simulink model "Dijkstra_Optimization_2"  (R2015b)
settings: Solver=FixedStepDiscrete  SolverMode=SingleTasking  StartTime=0.0  StopTime=10e-5  RelTol=1e-3
libraries: shlslibv1 x995
(part 1 of 6)
settings Model: synDspstartup=OK  Creator=irupawal  LastModifiedBy=vrames13
settings DataIOCC: SaveOutput=off  SignalLogging=off  SaveTime=off
settings OptimizationCC: DefaultParameterBehavior=Inlined
settings DebuggingCC: AlgebraicLoopMsg=error  InheritedTsInSrcMsg=none

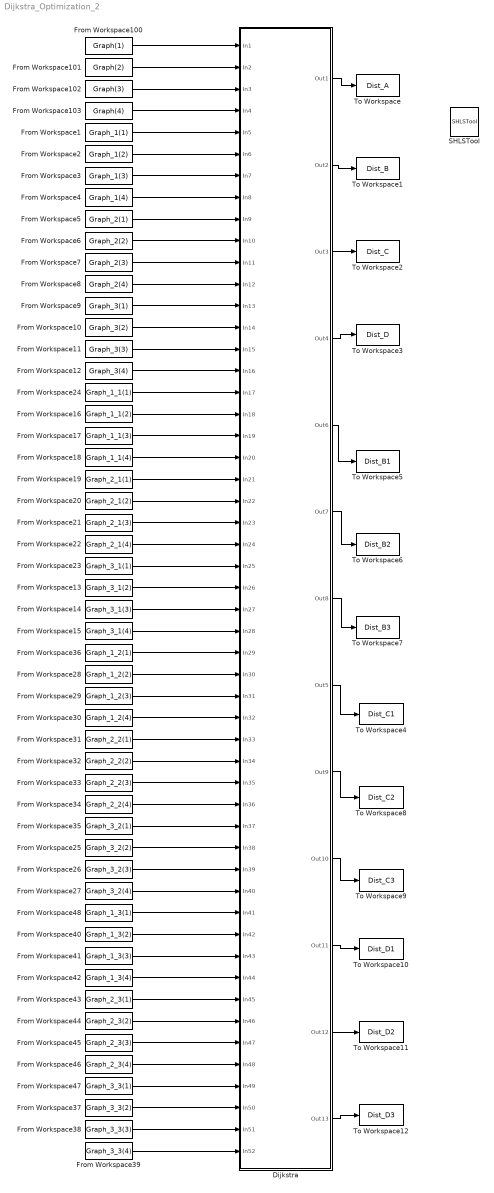
== system Dijkstra_Optimization_2 ==
  Dijkstra : Subsystem
  From Workspace1 : FromWorkspace  VariableName=Graph_1(1)  SampleTime=1/(16e6)  Interpolate=off  OutputAfterFinalValue=Holding final value
  From Workspace10 : FromWorkspace  VariableName=Graph_3(2)  SampleTime=1/(16e6)  Interpolate=off  OutputAfterFinalValue=Holding final value
  From Workspace100 : FromWorkspace  VariableName=Graph(1)  SampleTime=1/(16e6)  Interpolate=off  OutputAfterFinalValue=Holding final value
  From Workspace101 : FromWorkspace  VariableName=Graph(2)  SampleTime=1/(16e6)  Interpolate=off  OutputAfterFinalValue=Holding final value
  From Workspace102 : FromWorkspace  VariableName=Graph(3)  SampleTime=1/(16e6)  Interpolate=off  OutputAfterFinalValue=Holding final value
  From Workspace103 : FromWorkspace  VariableName=Graph(4)  SampleTime=1/(16e6)  Interpolate=off  OutputAfterFinalValue=Holding final value
  From Workspace11 : FromWorkspace  VariableName=Graph_3(3)  SampleTime=1/(16e6)  Interpolate=off  OutputAfterFinalValue=Holding final value
  From Workspace12 : FromWorkspace  VariableName=Graph_3(4)  SampleTime=1/(16e6)  Interpolate=off  OutputAfterFinalValue=Holding final value
  From Workspace13 : FromWorkspace  VariableName=Graph_3_1(2)  SampleTime=1/(16e6)  Interpolate=off  OutputAfterFinalValue=Holding final value
  From Workspace14 : FromWorkspace  VariableName=Graph_3_1(3)  SampleTime=1/(16e6)  Interpolate=off  OutputAfterFinalValue=Holding final value
  From Workspace15 : FromWorkspace  VariableName=Graph_3_1(4)  SampleTime=1/(16e6)  Interpolate=off  OutputAfterFinalValue=Holding final value
  From Workspace16 : FromWorkspace  VariableName=Graph_1_1(2)  SampleTime=1/(16e6)  Interpolate=off  OutputAfterFinalValue=Holding final value
  From Workspace17 : FromWorkspace  VariableName=Graph_1_1(3)  SampleTime=1/(16e6)  Interpolate=off  OutputAfterFinalValue=Holding final value
  From Workspace18 : FromWorkspace  VariableName=Graph_1_1(4)  SampleTime=1/(16e6)  Interpolate=off  OutputAfterFinalValue=Holding final value
  From Workspace19 : FromWorkspace  VariableName=Graph_2_1(1)  SampleTime=1/(16e6)  Interpolate=off  OutputAfterFinalValue=Holding final value
  From Workspace2 : FromWorkspace  VariableName=Graph_1(2)  SampleTime=1/(16e6)  Interpolate=off  OutputAfterFinalValue=Holding final value
  From Workspace20 : FromWorkspace  VariableName=Graph_2_1(2)  SampleTime=1/(16e6)  Interpolate=off  OutputAfterFinalValue=Holding final value
  From Workspace21 : FromWorkspace  VariableName=Graph_2_1(3)  SampleTime=1/(16e6)  Interpolate=off  OutputAfterFinalValue=Holding final value
  From Workspace22 : FromWorkspace  VariableName=Graph_2_1(4)  SampleTime=1/(16e6)  Interpolate=off  OutputAfterFinalValue=Holding final value
  From Workspace23 : FromWorkspace  VariableName=Graph_3_1(1)  SampleTime=1/(16e6)  Interpolate=off  OutputAfterFinalValue=Holding final value
  From Workspace24 : FromWorkspace  VariableName=Graph_1_1(1)  SampleTime=1/(16e6)  Interpolate=off  OutputAfterFinalValue=Holding final value
  From Workspace25 : FromWorkspace  VariableName=Graph_3_2(2)  SampleTime=1/(16e6)  Interpolate=off  OutputAfterFinalValue=Holding final value
  From Workspace26 : FromWorkspace  VariableName=Graph_3_2(3)  SampleTime=1/(16e6)  Interpolate=off  OutputAfterFinalValue=Holding final value
  From Workspace27 : FromWorkspace  VariableName=Graph_3_2(4)  SampleTime=1/(16e6)  Interpolate=off  OutputAfterFinalValue=Holding final value
  From Workspace28 : FromWorkspace  VariableName=Graph_1_2(2)  SampleTime=1/(16e6)  Interpolate=off  OutputAfterFinalValue=Holding final value
  From Workspace29 : FromWorkspace  VariableName=Graph_1_2(3)  SampleTime=1/(16e6)  Interpolate=off  OutputAfterFinalValue=Holding final value
  From Workspace3 : FromWorkspace  VariableName=Graph_1(3)  SampleTime=1/(16e6)  Interpolate=off  OutputAfterFinalValue=Holding final value
  From Workspace30 : FromWorkspace  VariableName=Graph_1_2(4)  SampleTime=1/(16e6)  Interpolate=off  OutputAfterFinalValue=Holding final value
  From Workspace31 : FromWorkspace  VariableName=Graph_2_2(1)  SampleTime=1/(16e6)  Interpolate=off  OutputAfterFinalValue=Holding final value
  From Workspace32 : FromWorkspace  VariableName=Graph_2_2(2)  SampleTime=1/(16e6)  Interpolate=off  OutputAfterFinalValue=Holding final value
  From Workspace33 : FromWorkspace  VariableName=Graph_2_2(3)  SampleTime=1/(16e6)  Interpolate=off  OutputAfterFinalValue=Holding final value
  From Workspace34 : FromWorkspace  VariableName=Graph_2_2(4)  SampleTime=1/(16e6)  Interpolate=off  OutputAfterFinalValue=Holding final value
  From Workspace35 : FromWorkspace  VariableName=Graph_3_2(1)  SampleTime=1/(16e6)  Interpolate=off  OutputAfterFinalValue=Holding final value
  From Workspace36 : FromWorkspace  VariableName=Graph_1_2(1)  SampleTime=1/(16e6)  Interpolate=off  OutputAfterFinalValue=Holding final value
  From Workspace37 : FromWorkspace  VariableName=Graph_3_3(2)  SampleTime=1/(16e6)  Interpolate=off  OutputAfterFinalValue=Holding final value
  From Workspace38 : FromWorkspace  VariableName=Graph_3_3(3)  SampleTime=1/(16e6)  Interpolate=off  OutputAfterFinalValue=Holding final value
  From Workspace39 : FromWorkspace  VariableName=Graph_3_3(4)  SampleTime=1/(16e6)  Interpolate=off  OutputAfterFinalValue=Holding final value
  From Workspace4 : FromWorkspace  VariableName=Graph_1(4)  SampleTime=1/(16e6)  Interpolate=off  OutputAfterFinalValue=Holding final value
  From Workspace40 : FromWorkspace  VariableName=Graph_1_3(2)  SampleTime=1/(16e6)  Interpolate=off  OutputAfterFinalValue=Holding final value
  From Workspace41 : FromWorkspace  VariableName=Graph_1_3(3)  SampleTime=1/(16e6)  Interpolate=off  OutputAfterFinalValue=Holding final value
  From Workspace42 : FromWorkspace  VariableName=Graph_1_3(4)  SampleTime=1/(16e6)  Interpolate=off  OutputAfterFinalValue=Holding final value
  From Workspace43 : FromWorkspace  VariableName=Graph_2_3(1)  SampleTime=1/(16e6)  Interpolate=off  OutputAfterFinalValue=Holding final value
  From Workspace44 : FromWorkspace  VariableName=Graph_2_3(2)  SampleTime=1/(16e6)  Interpolate=off  OutputAfterFinalValue=Holding final value
  From Workspace45 : FromWorkspace  VariableName=Graph_2_3(3)  SampleTime=1/(16e6)  Interpolate=off  OutputAfterFinalValue=Holding final value
  From Workspace46 : FromWorkspace  VariableName=Graph_2_3(4)  SampleTime=1/(16e6)  Interpolate=off  OutputAfterFinalValue=Holding final value
  From Workspace47 : FromWorkspace  VariableName=Graph_3_3(1)  SampleTime=1/(16e6)  Interpolate=off  OutputAfterFinalValue=Holding final value
  From Workspace48 : FromWorkspace  VariableName=Graph_1_3(1)  SampleTime=1/(16e6)  Interpolate=off  OutputAfterFinalValue=Holding final value
  From Workspace5 : FromWorkspace  VariableName=Graph_2(1)  SampleTime=1/(16e6)  Interpolate=off  OutputAfterFinalValue=Holding final value
  From Workspace6 : FromWorkspace  VariableName=Graph_2(2)  SampleTime=1/(16e6)  Interpolate=off  OutputAfterFinalValue=Holding final value
  From Workspace7 : FromWorkspace  VariableName=Graph_2(3)  SampleTime=1/(16e6)  Interpolate=off  OutputAfterFinalValue=Holding final value
  From Workspace8 : FromWorkspace  VariableName=Graph_2(4)  SampleTime=1/(16e6)  Interpolate=off  OutputAfterFinalValue=Holding final value
  From Workspace9 : FromWorkspace  VariableName=Graph_3(1)  SampleTime=1/(16e6)  Interpolate=off  OutputAfterFinalValue=Holding final value
  SHLSTool : shlslibv1/SHLSTool  synBlockType=tool  syn_dsp_mode=FPGA
  To Workspace : ToWorkspace  VariableName=Dist_A  SaveFormat=Timeseries  SampleTime=-1
  To Workspace1 : ToWorkspace  VariableName=Dist_B  SaveFormat=Timeseries  SampleTime=-1
  To Workspace10 : ToWorkspace  VariableName=Dist_D1  SaveFormat=Timeseries  SampleTime=-1
  To Workspace11 : ToWorkspace  VariableName=Dist_D2  SaveFormat=Timeseries  SampleTime=-1
  To Workspace12 : ToWorkspace  VariableName=Dist_D3  SaveFormat=Timeseries  SampleTime=-1
  To Workspace2 : ToWorkspace  VariableName=Dist_C  SaveFormat=Timeseries  SampleTime=-1
  To Workspace3 : ToWorkspace  VariableName=Dist_D  SaveFormat=Timeseries  SampleTime=-1
  To Workspace4 : ToWorkspace  VariableName=Dist_C1  SaveFormat=Timeseries  SampleTime=-1
  To Workspace5 : ToWorkspace  VariableName=Dist_B1  SaveFormat=Timeseries  SampleTime=-1
  To Workspace6 : ToWorkspace  VariableName=Dist_B2  SaveFormat=Timeseries  SampleTime=-1
  To Workspace7 : ToWorkspace  VariableName=Dist_B3  SaveFormat=Timeseries  SampleTime=-1
  To Workspace8 : ToWorkspace  VariableName=Dist_C2  SaveFormat=Timeseries  SampleTime=-1
  To Workspace9 : ToWorkspace  VariableName=Dist_C3  SaveFormat=Timeseries  SampleTime=-1
  wires:
  From Workspace100/1 -> Dijkstra/1(In1)
  From Workspace101/1 -> Dijkstra/2(In2)
  From Workspace102/1 -> Dijkstra/3(In3)
  From Workspace103/1 -> Dijkstra/4(In4)
  Dijkstra/1(Out1) -> To Workspace/1
  Dijkstra/2(Out2) -> To Workspace1/1
  Dijkstra/4(Out4) -> To Workspace3/1
  Dijkstra/3(Out3) -> To Workspace2/1
  From Workspace1/1 -> Dijkstra/5(In5)
  From Workspace2/1 -> Dijkstra/6(In6)
  From Workspace3/1 -> Dijkstra/7(In7)
  From Workspace4/1 -> Dijkstra/8(In8)
  From Workspace5/1 -> Dijkstra/9(In9)
  From Workspace6/1 -> Dijkstra/10(In10)
  From Workspace7/1 -> Dijkstra/11(In11)
  From Workspace8/1 -> Dijkstra/12(In12)
  From Workspace9/1 -> Dijkstra/13(In13)
  From Workspace10/1 -> Dijkstra/14(In14)
  From Workspace11/1 -> Dijkstra/15(In15)
  From Workspace12/1 -> Dijkstra/16(In16)
  Dijkstra/5(Out6) -> To Workspace5/1
  Dijkstra/6(Out7) -> To Workspace6/1
  Dijkstra/7(Out8) -> To Workspace7/1
  From Workspace16/1 -> Dijkstra/18(In18)
  From Workspace17/1 -> Dijkstra/19(In19)
  From Workspace18/1 -> Dijkstra/20(In20)
  From Workspace19/1 -> Dijkstra/21(In21)
  From Workspace20/1 -> Dijkstra/22(In22)
  From Workspace21/1 -> Dijkstra/23(In23)
  From Workspace22/1 -> Dijkstra/24(In24)
  From Workspace23/1 -> Dijkstra/25(In25)
  From Workspace13/1 -> Dijkstra/26(In26)
  From Workspace14/1 -> Dijkstra/27(In27)
  From Workspace15/1 -> Dijkstra/28(In28)
  From Workspace24/1 -> Dijkstra/17(In17)
  Dijkstra/8(Out5) -> To Workspace4/1
  Dijkstra/9(Out9) -> To Workspace8/1
  Dijkstra/10(Out10) -> To Workspace9/1
  Dijkstra/11(Out11) -> To Workspace10/1
  Dijkstra/12(Out12) -> To Workspace11/1
  Dijkstra/13(Out13) -> To Workspace12/1
  From Workspace36/1 -> Dijkstra/29(In29)
  From Workspace28/1 -> Dijkstra/30(In30)
  From Workspace29/1 -> Dijkstra/31(In31)
  From Workspace30/1 -> Dijkstra/32(In32)
  From Workspace31/1 -> Dijkstra/33(In33)
  From Workspace32/1 -> Dijkstra/34(In34)
  From Workspace33/1 -> Dijkstra/35(In35)
  From Workspace34/1 -> Dijkstra/36(In36)
  From Workspace35/1 -> Dijkstra/37(In37)
  From Workspace25/1 -> Dijkstra/38(In38)
  From Workspace26/1 -> Dijkstra/39(In39)
  From Workspace27/1 -> Dijkstra/40(In40)
  From Workspace48/1 -> Dijkstra/41(In41)
  From Workspace40/1 -> Dijkstra/42(In42)
  From Workspace41/1 -> Dijkstra/43(In43)
  From Workspace42/1 -> Dijkstra/44(In44)
  From Workspace43/1 -> Dijkstra/45(In45)
  From Workspace44/1 -> Dijkstra/46(In46)
  From Workspace45/1 -> Dijkstra/47(In47)
  From Workspace46/1 -> Dijkstra/48(In48)
  From Workspace47/1 -> Dijkstra/49(In49)
  From Workspace37/1 -> Dijkstra/50(In50)
  From Workspace38/1 -> Dijkstra/51(In51)
  From Workspace39/1 -> Dijkstra/52(In52)

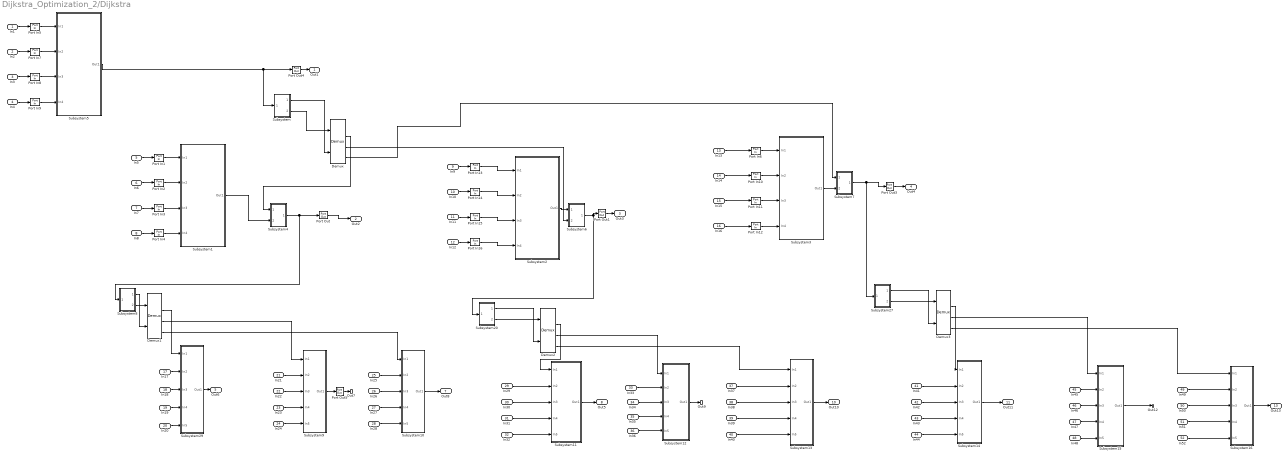
== system Dijkstra_Optimization_2/Dijkstra ==
  In1 : Inport
  In2 : Inport  Port=2
  In3 : Inport  Port=3
  In4 : Inport  Port=4
  In5 : Inport  Port=5
  In6 : Inport  Port=6
  In7 : Inport  Port=7
  In8 : Inport  Port=8
  In9 : Inport  Port=9
  In10 : Inport  Port=10
  In11 : Inport  Port=11
  In12 : Inport  Port=12
  In13 : Inport  Port=13
  In14 : Inport  Port=14
  In15 : Inport  Port=15
  In16 : Inport  Port=16
  In17 : Inport  Port=17
  In18 : Inport  Port=18
  In19 : Inport  Port=19
  In20 : Inport  Port=20
  In21 : Inport  Port=21
  In22 : Inport  Port=22
  In23 : Inport  Port=23
  In24 : Inport  Port=24
  In25 : Inport  Port=25
  In26 : Inport  Port=26
  In27 : Inport  Port=27
  In28 : Inport  Port=28
  In29 : Inport  Port=29
  In30 : Inport  Port=30
  In31 : Inport  Port=31
  In32 : Inport  Port=32
  In33 : Inport  Port=33
  In34 : Inport  Port=34
  In35 : Inport  Port=35
  In36 : Inport  Port=36
  In37 : Inport  Port=37
  In38 : Inport  Port=38
  In39 : Inport  Port=39
  In40 : Inport  Port=40
  In41 : Inport  Port=41
  In42 : Inport  Port=42
  In43 : Inport  Port=43
  In44 : Inport  Port=44
  In45 : Inport  Port=45
  In46 : Inport  Port=46
  In47 : Inport  Port=47
  In48 : Inport  Port=48
  In49 : Inport  Port=49
  In50 : Inport  Port=50
  In51 : Inport  Port=51
  In52 : Inport  Port=52
  Demux{,1..3} (4 alike) : shlslibv1/Signal Operations/Demux  syn_out_nb=4  syn_out_latch=off  synBlockType=primitive  synLatency=0  synBlockId=18
  Port In{1..16} (16 alike) : shlslibv1/Ports & Subsystems/Port In  syn_out_wl=50  syn_out_fl=0  syn_out_dt=unsigned  syn_out_st=1/(4e6)  syn_capture=on  syn_register=on  syn_out_sat=off  syn_out_rnd=on  synBlockType=port  synLatency=1  synBlockId=0
  Port Out{,1,3..5} (5 alike) : shlslibv1/Ports & Subsystems/Port Out  syn_capture=off  syn_register=on  synBlockType=port  synLatency=1  synBlockId=1
  Subsystem : Subsystem
  Subsystem1 : Subsystem
  Subsystem10 : Subsystem
  Subsystem11 : Subsystem
  Subsystem12 : Subsystem
  Subsystem13 : Subsystem
  Subsystem14 : Subsystem
  Subsystem15 : Subsystem
  Subsystem16 : Subsystem
  Subsystem2 : Subsystem
  Subsystem20 : Subsystem
  Subsystem27 : Subsystem
  Subsystem29 : Subsystem
  Subsystem3 : Subsystem
  Subsystem4 : Subsystem
  Subsystem5 : Subsystem
  Subsystem6 : Subsystem
  Subsystem7 : Subsystem
  Subsystem8 : Subsystem
  Subsystem9 : Subsystem
  Out1 : Outport
  Out2 : Outport  Port=2
  Out3 : Outport  Port=3
  Out4 : Outport  Port=4
  Out6 : Outport  Port=5
  Out7 : Outport  Port=6
  Out8 : Outport  Port=7
  Out5 : Outport  Port=8
  Out9 : Outport  Port=9
  Out10 : Outport  Port=10
  Out11 : Outport  Port=11
  Out12 : Outport  Port=12
  Out13 : Outport  Port=13
  wires:
  Port In11/1 -> Subsystem3/3(In3)
  In6/1 -> Port In2/1
  In7/1 -> Port In3/1
  In8/1 -> Port In4/1
  Port In1/1 -> Subsystem1/1(In1)
  Port In3/1 -> Subsystem1/3(In3)
  In3/1 -> Port In8/1
  In9/1 -> Port In13/1
  In10/1 -> Port In14/1
  In11/1 -> Port In15/1
  In12/1 -> Port In16/1
  Port In14/1 -> Subsystem2/2(In2)
  Port In13/1 -> Subsystem2/1(In1)
  Port In16/1 -> Subsystem2/4(In4)
  Port In15/1 -> Subsystem2/3(In3)
  In13/1 -> Port In6/1
  In14/1 -> Port In10/1
  In15/1 -> Port In11/1
  In16/1 -> Port In12/1
  Port In10/1 -> Subsystem3/2(In2)
  Port In6/1 -> Subsystem3/1(In1)
  Port In12/1 -> Subsystem3/4(In4)
  In1/1 -> Port In5/1
  Port In8/1 -> Subsystem5/3(In3)
  In4/1 -> Port In9/1
  In5/1 -> Port In1/1
  In2/1 -> Port In7/1
  Port In5/1 -> Subsystem5/1(In1)
  Port In2/1 -> Subsystem1/2(In2)
  Port In4/1 -> Subsystem1/4(In4)
  Port In7/1 -> Subsystem5/2(In2)
  Port In9/1 -> Subsystem5/4(In4)
  Subsystem5/1(Out1) -> Port Out4/1, Subsystem/1(In1)
  Port Out4/1 -> Out1/1
  Subsystem/1(Out1) -> Demux/2
  Subsystem/2(Out2) -> Demux/1
  Demux/2 -> Subsystem4/1(In1)
  Subsystem1/1(Out1) -> Subsystem4/2(In2)
  Subsystem2/1(Out1) -> Subsystem6/1(In1)
  Demux/3 -> Subsystem6/2(In2)
  Demux/4 -> Subsystem7/1(In1)
  Subsystem3/1(Out1) -> Subsystem7/2(In2)
  Subsystem7/1(Out1) -> Subsystem27/1(In1), Port Out3/1
  Subsystem4/1(Out1) -> Port Out/1, Subsystem8/1(In1)
  Subsystem8/1(Out1) -> Demux1/2
  Subsystem8/2(Out2) -> Demux1/1
  Port Out/1 -> Out2/1
  Port Out1/1 -> Out3/1
  Port Out3/1 -> Out4/1
  Port Out5/1 -> Out7/1
  Subsystem6/1(Out1) -> Port Out1/1, Subsystem20/1(In1)
  Subsystem20/1(Out1) -> Demux2/2
  Subsystem20/2(Out2) -> Demux2/1
  Subsystem27/1(Out1) -> Demux3/2
  Subsystem27/2(Out2) -> Demux3/1
  Demux1/2 -> Subsystem29/1(In1)
  In17/1 -> Subsystem29/2(In2)
  In18/1 -> Subsystem29/3(In3)
  In19/1 -> Subsystem29/4(In4)
  In20/1 -> Subsystem29/5(In5)
  Subsystem29/1(Out1) -> Out6/1
  Demux1/3 -> Subsystem9/1(In1)
  In21/1 -> Subsystem9/2(In2)
  In22/1 -> Subsystem9/3(In3)
  In23/1 -> Subsystem9/4(In4)
  In24/1 -> Subsystem9/5(In5)
  Subsystem9/1(Out1) -> Port Out5/1
  Demux1/4 -> Subsystem10/1(In1)
  In25/1 -> Subsystem10/2(In2)
  In26/1 -> Subsystem10/3(In3)
  In27/1 -> Subsystem10/4(In4)
  In28/1 -> Subsystem10/5(In5)
  Subsystem10/1(Out1) -> Out8/1
  Demux2/2 -> Subsystem11/1(In1)
  In29/1 -> Subsystem11/2(In2)
  In30/1 -> Subsystem11/3(In3)
  In31/1 -> Subsystem11/4(In4)
  In32/1 -> Subsystem11/5(In5)
  Subsystem11/1(Out1) -> Out5/1
  Demux2/3 -> Subsystem12/1(In1)
  In33/1 -> Subsystem12/2(In2)
  In34/1 -> Subsystem12/3(In3)
  In35/1 -> Subsystem12/4(In4)
  In36/1 -> Subsystem12/5(In5)
  Subsystem12/1(Out1) -> Out9/1
  Demux2/4 -> Subsystem13/1(In1)
  In37/1 -> Subsystem13/2(In2)
  In38/1 -> Subsystem13/3(In3)
  In39/1 -> Subsystem13/4(In4)
  In40/1 -> Subsystem13/5(In5)
  Subsystem13/1(Out1) -> Out10/1
  Demux3/2 -> Subsystem14/1(In1)
  In41/1 -> Subsystem14/2(In2)
  In42/1 -> Subsystem14/3(In3)
  In43/1 -> Subsystem14/4(In4)
  In44/1 -> Subsystem14/5(In5)
  Subsystem14/1(Out1) -> Out11/1
  Demux3/3 -> Subsystem15/1(In1)
  In45/1 -> Subsystem15/2(In2)
  In46/1 -> Subsystem15/3(In3)
  In47/1 -> Subsystem15/4(In4)
  In48/1 -> Subsystem15/5(In5)
  Subsystem15/1(Out1) -> Out12/1
  Demux3/4 -> Subsystem16/1(In1)
  In49/1 -> Subsystem16/2(In2)
  In50/1 -> Subsystem16/3(In3)
  In51/1 -> Subsystem16/4(In4)
  In52/1 -> Subsystem16/5(In5)
  Subsystem16/1(Out1) -> Out13/1

== system Dijkstra_Optimization_2/Dijkstra/Subsystem ==
  In1 : Inport
  Constant3 : shlslibv1/Sources/Constant  syn_cst_val=1  syn_cst_format=Automatic  syn_cst_wl=1  syn_cst_fl=0  syn_cst_dt=unsigned  syn_cst_rnd=on  syn_cst_st=-1  synBlockType=primitive  synLatency=0  synBlockId=15
  Switch6 : shlslibv1/Signal Operations/Switch  switchCriteria=u2 == Threshold  switchThresh=0  synBlockType=custom  synLatency=0
  dist8 : shlslibv1/Sources/Sequence  syn_seq_vec=[0 1 2 3]  syn_seq_wl=4  syn_seq_fl=0  syn_seq_dt=unsigned  syn_rst_port=off  syn_en_port=off  syn_seq_st=1/(4e6)  synBlockType=custom  synLatency=1
  min1 : shlslibv1/Memories/Delay  syn_delay_val=26  synBlockType=primitive  synLatency=26  synBlockId=104
  min12 : shlslibv1/Memories/Delay  syn_delay_val=28  synBlockType=primitive  synLatency=28  synBlockId=104
  Out1 : Outport
  Out2 : Outport  Port=2
  wires:
  In1/1 -> Switch6/3
  Constant3/1 -> min12/1
  min12/1 -> Switch6/1, Switch6/2
  Switch6/1 -> Out1/1
  min1/1 -> Out2/1
  dist8/1 -> min1/1

== system Dijkstra_Optimization_2/Dijkstra/Subsystem1 ==
  In1 : Inport
  In2 : Inport  Port=2
  In3 : Inport  Port=3
  In4 : Inport  Port=4
  Delay : Subsystem
  Input : Subsystem
  Min_index : Subsystem
  initial : Subsystem
  min_distance : Subsystem
  Out1 : Outport
  wires:
  min_distance/2(Out2) -> initial/3(In3)
  Input/1(Out1) -> min_distance/5(In5)
  min_distance/1(Out1) -> initial/2(In2)
  Input/2(Out2) -> min_distance/6(In6)
  Min_index/1(min_sub) -> Delay/1(In1)
  In4/1 -> Input/4(In4)
  initial/1(Out1) -> Min_index/1(dout_sub), Out1/1
  initial/3(Out3) -> min_distance/1(In1)
  In3/1 -> Input/3(In3)
  In2/1 -> Input/2(In2)
  initial/4(Out4) -> min_distance/4(In4)
  initial/2(Out2) -> Min_index/2(doutsp_sub)
  Min_index/2(min_index_sub) -> Delay/2(In2), initial/1(In1)
  Delay/2(Out2) -> min_distance/3(In3)
  Delay/1(Out1) -> min_distance/2(In2)
  In1/1 -> Input/1(In1)
  Input/3(Out3) -> min_distance/7(In7)
  Input/4(Out4) -> min_distance/8(In8)

== system Dijkstra_Optimization_2/Dijkstra/Subsystem10 ==
  In1 : Inport
  In2 : Inport  Port=2
  In3 : Inport  Port=3
  In4 : Inport  Port=4
  In5 : Inport  Port=5
  Port In{18..20,28} (4 alike) : shlslibv1/Ports & Subsystems/Port In  syn_out_wl=50  syn_out_fl=0  syn_out_dt=unsigned  syn_out_st=1/(4e6)  syn_capture=on  syn_register=on  syn_out_sat=off  syn_out_rnd=on  synBlockType=port  synLatency=1  synBlockId=0
  Port Out6 : shlslibv1/Ports & Subsystems/Port Out  syn_capture=off  syn_register=on  synBlockType=port  synLatency=1  synBlockId=1
  Subsystem11 : Subsystem
  Subsystem14 : Subsystem
  Out1 : Outport
  wires:
  In3/1 -> Port In18/1
  In2/1 -> Port In28/1
  Port In20/1 -> Subsystem11/4(In4)
  In5/1 -> Port In20/1
  In1/1 -> Subsystem14/1(In1)
  Subsystem11/1(Out1) -> Subsystem14/2(In2)
  Subsystem14/1(Out1) -> Port Out6/1
  Port In28/1 -> Subsystem11/1(In1)
  In4/1 -> Port In19/1
  Port In18/1 -> Subsystem11/2(In2)
  Port In19/1 -> Subsystem11/3(In3)
  Port Out6/1 -> Out1/1

== system Dijkstra_Optimization_2/Dijkstra/Subsystem11 ==
  In1 : Inport
  In2 : Inport  Port=2
  In3 : Inport  Port=3
  In4 : Inport  Port=4
  In5 : Inport  Port=5
  Port In{29,37..39} (4 alike) : shlslibv1/Ports & Subsystems/Port In  syn_out_wl=50  syn_out_fl=0  syn_out_dt=unsigned  syn_out_st=1/(4e6)  syn_capture=on  syn_register=on  syn_out_sat=off  syn_out_rnd=on  synBlockType=port  synLatency=1  synBlockId=0
  Port Out7 : shlslibv1/Ports & Subsystems/Port Out  syn_capture=off  syn_register=on  synBlockType=port  synLatency=1  synBlockId=1
  Subsystem17 : Subsystem
  Subsystem21 : Subsystem
  Out1 : Outport
  wires:
  In4/1 -> Port In38/1
  Port In29/1 -> Subsystem21/1(In1)
  In5/1 -> Port In39/1
  Port In38/1 -> Subsystem21/3(In3)
  In3/1 -> Port In37/1
  In1/1 -> Subsystem17/1(In1)
  Port In39/1 -> Subsystem21/4(In4)
  Port In37/1 -> Subsystem21/2(In2)
  In2/1 -> Port In29/1
  Subsystem21/1(Out1) -> Subsystem17/2(In2)
  Subsystem17/1(Out1) -> Port Out7/1
  Port Out7/1 -> Out1/1

== system Dijkstra_Optimization_2/Dijkstra/Subsystem12 ==
  In1 : Inport
  In2 : Inport  Port=2
  In3 : Inport  Port=3
  In4 : Inport  Port=4
  In5 : Inport  Port=5
  Port In{33..36} (4 alike) : shlslibv1/Ports & Subsystems/Port In  syn_out_wl=50  syn_out_fl=0  syn_out_dt=unsigned  syn_out_st=1/(4e6)  syn_capture=on  syn_register=on  syn_out_sat=off  syn_out_rnd=on  synBlockType=port  synLatency=1  synBlockId=0
  Port Out8 : shlslibv1/Ports & Subsystems/Port Out  syn_capture=off  syn_register=on  synBlockType=port  synLatency=1  synBlockId=1
  Subsystem15 : Subsystem
  Subsystem18 : Subsystem
  Out1 : Outport
  wires:
  In4/1 -> Port In35/1
  Port In35/1 -> Subsystem15/3(In3)
  Subsystem18/1(Out1) -> Port Out8/1
  In3/1 -> Port In34/1
  Port In36/1 -> Subsystem15/4(In4)
  Port In33/1 -> Subsystem15/1(In1)
  In5/1 -> Port In36/1
  In1/1 -> Subsystem18/2(In2)
  Port In34/1 -> Subsystem15/2(In2)
  In2/1 -> Port In33/1
  Port Out8/1 -> Out1/1
  Subsystem15/1(Out1) -> Subsystem18/1(In1)

== system Dijkstra_Optimization_2/Dijkstra/Subsystem13 ==
  In1 : Inport
  In2 : Inport  Port=2
  In3 : Inport  Port=3
  In4 : Inport  Port=4
  In5 : Inport  Port=5
  Port In{30..32,40} (4 alike) : shlslibv1/Ports & Subsystems/Port In  syn_out_wl=50  syn_out_fl=0  syn_out_dt=unsigned  syn_out_st=1/(4e6)  syn_capture=on  syn_register=on  syn_out_sat=off  syn_out_rnd=on  synBlockType=port  synLatency=1  synBlockId=0
  Port Out9 : shlslibv1/Ports & Subsystems/Port Out  syn_capture=off  syn_register=on  synBlockType=port  synLatency=1  synBlockId=1
  Subsystem16 : Subsystem
  Subsystem19 : Subsystem
  Out1 : Outport
  wires:
  Subsystem16/1(Out1) -> Subsystem19/2(In2)
  In5/1 -> Port In32/1
  In1/1 -> Subsystem19/1(In1)
  Subsystem19/1(Out1) -> Port Out9/1
  In4/1 -> Port In31/1
  In2/1 -> Port In40/1
  Port Out9/1 -> Out1/1
  Port In40/1 -> Subsystem16/1(In1)
  Port In30/1 -> Subsystem16/2(In2)
  In3/1 -> Port In30/1
  Port In31/1 -> Subsystem16/3(In3)
  Port In32/1 -> Subsystem16/4(In4)

== system Dijkstra_Optimization_2/Dijkstra/Subsystem14 ==
  In1 : Inport
  In2 : Inport  Port=2
  In3 : Inport  Port=3
  In4 : Inport  Port=4
  In5 : Inport  Port=5
  Port In{41,49..51} (4 alike) : shlslibv1/Ports & Subsystems/Port In  syn_out_wl=50  syn_out_fl=0  syn_out_dt=unsigned  syn_out_st=1/(4e6)  syn_capture=on  syn_register=on  syn_out_sat=off  syn_out_rnd=on  synBlockType=port  synLatency=1  synBlockId=0
  Port Out10 : shlslibv1/Ports & Subsystems/Port Out  syn_capture=off  syn_register=on  synBlockType=port  synLatency=1  synBlockId=1
  Subsystem24 : Subsystem
  Subsystem28 : Subsystem
  Out1 : Outport
  wires:
  Subsystem28/1(Out1) -> Subsystem24/2(In2)
  Port In49/1 -> Subsystem28/2(In2)
  Port In51/1 -> Subsystem28/4(In4)
  Port In41/1 -> Subsystem28/1(In1)
  In1/1 -> Subsystem24/1(In1)
  In5/1 -> Port In51/1
  In3/1 -> Port In49/1
  Subsystem24/1(Out1) -> Port Out10/1
  Port In50/1 -> Subsystem28/3(In3)
  In4/1 -> Port In50/1
  Port Out10/1 -> Out1/1
  In2/1 -> Port In41/1

== system Dijkstra_Optimization_2/Dijkstra/Subsystem15 ==
  In1 : Inport
  In2 : Inport  Port=2
  In3 : Inport  Port=3
  In4 : Inport  Port=4
  In5 : Inport  Port=5
  Port In{45..48} (4 alike) : shlslibv1/Ports & Subsystems/Port In  syn_out_wl=50  syn_out_fl=0  syn_out_dt=unsigned  syn_out_st=1/(4e6)  syn_capture=on  syn_register=on  syn_out_sat=off  syn_out_rnd=on  synBlockType=port  synLatency=1  synBlockId=0
  Port Out11 : shlslibv1/Ports & Subsystems/Port Out  syn_capture=off  syn_register=on  synBlockType=port  synLatency=1  synBlockId=1
  Subsystem22 : Subsystem
  Subsystem25 : Subsystem
  Out1 : Outport
  wires:
  Port In45/1 -> Subsystem22/1(In1)
  In3/1 -> Port In46/1
  Subsystem25/1(Out1) -> Port Out11/1
  In1/1 -> Subsystem25/2(In2)
  In4/1 -> Port In47/1
  Port In48/1 -> Subsystem22/4(In4)
  Subsystem22/1(Out1) -> Subsystem25/1(In1)
  Port In46/1 -> Subsystem22/2(In2)
  Port Out11/1 -> Out1/1
  In5/1 -> Port In48/1
  Port In47/1 -> Subsystem22/3(In3)
  In2/1 -> Port In45/1

== system Dijkstra_Optimization_2/Dijkstra/Subsystem16 ==
  In1 : Inport
  In2 : Inport  Port=2
  In3 : Inport  Port=3
  In4 : Inport  Port=4
  In5 : Inport  Port=5
  Port In{42..44,52} (4 alike) : shlslibv1/Ports & Subsystems/Port In  syn_out_wl=50  syn_out_fl=0  syn_out_dt=unsigned  syn_out_st=1/(4e6)  syn_capture=on  syn_register=on  syn_out_sat=off  syn_out_rnd=on  synBlockType=port  synLatency=1  synBlockId=0
  Port Out12 : shlslibv1/Ports & Subsystems/Port Out  syn_capture=off  syn_register=on  synBlockType=port  synLatency=1  synBlockId=1
  Subsystem23 : Subsystem
  Subsystem26 : Subsystem
  Out1 : Outport
  wires:
  Port In42/1 -> Subsystem23/2(In2)
  Port In44/1 -> Subsystem23/4(In4)
  In4/1 -> Port In43/1
  Subsystem26/1(Out1) -> Port Out12/1
  Port Out12/1 -> Out1/1
  In5/1 -> Port In44/1
  Port In43/1 -> Subsystem23/3(In3)
  In1/1 -> Subsystem26/1(In1)
  In3/1 -> Port In42/1
  In2/1 -> Port In52/1
  Port In52/1 -> Subsystem23/1(In1)
  Subsystem23/1(Out1) -> Subsystem26/2(In2)

== system Dijkstra_Optimization_2/Dijkstra/Subsystem2 ==
  In1 : Inport
  In2 : Inport  Port=2
  In3 : Inport  Port=3
  In4 : Inport  Port=4
  Delay : Subsystem
  Input : Subsystem
  Min_index : Subsystem
  initial : Subsystem
  min_distance : Subsystem
  Out1 : Outport
  wires:
  min_distance/2(Out2) -> initial/3(In3)
  Input/1(Out1) -> min_distance/5(In5)
  min_distance/1(Out1) -> initial/2(In2)
  Input/2(Out2) -> min_distance/6(In6)
  Min_index/1(min_sub) -> Delay/1(In1)
  In4/1 -> Input/4(In4)
  initial/1(Out1) -> Min_index/1(dout_sub), Out1/1
  initial/3(Out3) -> min_distance/1(In1)
  In3/1 -> Input/3(In3)
  In2/1 -> Input/2(In2)
  initial/4(Out4) -> min_distance/4(In4)
  initial/2(Out2) -> Min_index/2(doutsp_sub)
  Min_index/2(min_index_sub) -> Delay/2(In2), initial/1(In1)
  Delay/2(Out2) -> min_distance/3(In3)
  Delay/1(Out1) -> min_distance/2(In2)
  In1/1 -> Input/1(In1)
  Input/3(Out3) -> min_distance/7(In7)
  Input/4(Out4) -> min_distance/8(In8)

== system Dijkstra_Optimization_2/Dijkstra/Subsystem20 ==
  In1 : Inport
  Constant3 : shlslibv1/Sources/Constant  syn_cst_val=1  syn_cst_format=Automatic  syn_cst_wl=1  syn_cst_fl=0  syn_cst_dt=unsigned  syn_cst_rnd=on  syn_cst_st=-1  synBlockType=primitive  synLatency=0  synBlockId=15
  Switch6 : shlslibv1/Signal Operations/Switch  switchCriteria=u2 == Threshold  switchThresh=0  synBlockType=custom  synLatency=0
  dist8 : shlslibv1/Sources/Sequence  syn_seq_vec=[0 1 2 3]  syn_seq_wl=4  syn_seq_fl=0  syn_seq_dt=unsigned  syn_rst_port=off  syn_en_port=off  syn_seq_st=1/(4e6)  synBlockType=custom  synLatency=1
  min1 : shlslibv1/Memories/Delay  syn_delay_val=31  synBlockType=primitive  synLatency=31  synBlockId=104
  min12 : shlslibv1/Memories/Delay  syn_delay_val=34  synBlockType=primitive  synLatency=34  synBlockId=104
  Out1 : Outport
  Out2 : Outport  Port=2
  wires:
  Constant3/1 -> min12/1
  min12/1 -> Switch6/2, Switch6/1
  Switch6/1 -> Out1/1
  min1/1 -> Out2/1
  dist8/1 -> min1/1
  In1/1 -> Switch6/3

== system Dijkstra_Optimization_2/Dijkstra/Subsystem27 ==
  In1 : Inport
  Constant3 : shlslibv1/Sources/Constant  syn_cst_val=1  syn_cst_format=Automatic  syn_cst_wl=1  syn_cst_fl=0  syn_cst_dt=unsigned  syn_cst_rnd=on  syn_cst_st=-1  synBlockType=primitive  synLatency=0  synBlockId=15
  Switch6 : shlslibv1/Signal Operations/Switch  switchCriteria=u2 == Threshold  switchThresh=0  synBlockType=custom  synLatency=0
  dist8 : shlslibv1/Sources/Sequence  syn_seq_vec=[0 1 2 3]  syn_seq_wl=4  syn_seq_fl=0  syn_seq_dt=unsigned  syn_rst_port=off  syn_en_port=off  syn_seq_st=1/(4e6)  synBlockType=custom  synLatency=1
  min1 : shlslibv1/Memories/Delay  syn_delay_val=32  synBlockType=primitive  synLatency=32  synBlockId=104
  min12 : shlslibv1/Memories/Delay  syn_delay_val=35  synBlockType=primitive  synLatency=35  synBlockId=104
  Out1 : Outport
  Out2 : Outport  Port=2
  wires:
  Constant3/1 -> min12/1
  min12/1 -> Switch6/2, Switch6/1
  Switch6/1 -> Out1/1
  min1/1 -> Out2/1
  dist8/1 -> min1/1
  In1/1 -> Switch6/3

== system Dijkstra_Optimization_2/Dijkstra/Subsystem29 ==
  In1 : Inport
  In2 : Inport  Port=2
  In3 : Inport  Port=3
  In4 : Inport  Port=4
  In5 : Inport  Port=5
  Port In{17,25..27} (4 alike) : shlslibv1/Ports & Subsystems/Port In  syn_out_wl=50  syn_out_fl=0  syn_out_dt=unsigned  syn_out_st=1/(4e6)  syn_capture=on  syn_register=on  syn_out_sat=off  syn_out_rnd=on  synBlockType=port  synLatency=1  synBlockId=0
  Port Out2 : shlslibv1/Ports & Subsystems/Port Out  syn_capture=off  syn_register=on  synBlockType=port  synLatency=1  synBlockId=1
  Subsystem12 : Subsystem
  Subsystem9 : Subsystem
  To Workspace : ToWorkspace  VariableName=simout  SaveFormat=Timeseries  SampleTime=-1
  To Workspace1 : ToWorkspace  VariableName=simout1  SaveFormat=Timeseries  SampleTime=-1
  Out1 : Outport
  wires:
  In3/1 -> Port In25/1
  Subsystem12/1(Out1) -> Port Out2/1
  Subsystem9/1(Out1) -> To Workspace/1, Subsystem12/2(In2)
  In2/1 -> Port In17/1
  Port In27/1 -> Subsystem9/4(In4)
  In4/1 -> Port In26/1
  Port In25/1 -> Subsystem9/2(In2)
  Port In26/1 -> Subsystem9/3(In3)
  Port In17/1 -> Subsystem9/1(In1)
  Port Out2/1 -> Out1/1
  In5/1 -> Port In27/1
  In1/1 -> To Workspace1/1, Subsystem12/1(In1)

== system Dijkstra_Optimization_2/Dijkstra/Subsystem3 ==
  In1 : Inport
  In2 : Inport  Port=2
  In3 : Inport  Port=3
  In4 : Inport  Port=4
  Delay : Subsystem
  Input : Subsystem
  Min_index : Subsystem
  initial : Subsystem
  min_distance : Subsystem
  Out1 : Outport
  wires:
  min_distance/2(Out2) -> initial/3(In3)
  Input/1(Out1) -> min_distance/5(In5)
  min_distance/1(Out1) -> initial/2(In2)
  Input/2(Out2) -> min_distance/6(In6)
  Min_index/1(min_sub) -> Delay/1(In1)
  In4/1 -> Input/4(In4)
  initial/1(Out1) -> Min_index/1(dout_sub), Out1/1
  initial/3(Out3) -> min_distance/1(In1)
  In3/1 -> Input/3(In3)
  In2/1 -> Input/2(In2)
  initial/4(Out4) -> min_distance/4(In4)
  initial/2(Out2) -> Min_index/2(doutsp_sub)
  Min_index/2(min_index_sub) -> Delay/2(In2), initial/1(In1)
  Delay/2(Out2) -> min_distance/3(In3)
  Delay/1(Out1) -> min_distance/2(In2)
  In1/1 -> Input/1(In1)
  Input/3(Out3) -> min_distance/7(In7)
  Input/4(Out4) -> min_distance/8(In8)

== system Dijkstra_Optimization_2/Dijkstra/Subsystem4 ==
  In1 : Inport
  In2 : Inport  Port=2
  Add1 : shlslibv1/Math Functions/Add  syn_add_opr=++  syn_out_f=Full Precision  syn_out_wl=16  syn_out_fl=8  syn_out_dt=signed  syn_out_sat=off  syn_out_rnd=Floor (Truncate)  synBlockType=primitive  synLatency=0  synBlockId=96  syn_sum_of_rows=off  syn_inh_port=off  syn_inh_st=on  syn_inh_stf=1  syn_en_pipe=off  syn_pipe_stg=syn_max_pipeline  syn_flow_ctrl=off
  Constant1 : shlslibv1/Sources/Constant  syn_cst_val=1  syn_cst_format=Automatic  syn_cst_wl=1  syn_cst_fl=0  syn_cst_dt=unsigned  syn_cst_rnd=on  syn_cst_st=-1  synBlockType=primitive  synLatency=0  synBlockId=15
  Switch10 : shlslibv1/Signal Operations/Switch  switchCriteria=u2 != Threshold  switchThresh=0  synBlockType=custom  synLatency=0
  min2 : shlslibv1/Memories/Delay  syn_delay_val=1  synBlockType=primitive  synLatency=1  synBlockId=104
  min3 : shlslibv1/Memories/Delay  syn_delay_val=29  synBlockType=primitive  synLatency=29  synBlockId=104
  Out1 : Outport
  wires:
  Add1/1 -> Out1/1
  In2/1 -> Add1/2
  min2/1 -> Switch10/1
  Switch10/1 -> min2/1, Add1/1
  min3/1 -> Switch10/2
  Constant1/1 -> min3/1
  In1/1 -> Switch10/3

== system Dijkstra_Optimization_2/Dijkstra/Subsystem5 ==
  In1 : Inport
  In2 : Inport  Port=2
  In3 : Inport  Port=3
  In4 : Inport  Port=4
  Delay : Subsystem
  Input : Subsystem
  Min_index : Subsystem
  initial : Subsystem
  min_distance : Subsystem
  Out1 : Outport
  wires:
  min_distance/2(Out2) -> initial/3(In3)
  Input/1(Out1) -> min_distance/5(In5)
  min_distance/1(Out1) -> initial/2(In2)
  Input/2(Out2) -> min_distance/6(In6)
  Min_index/1(min_sub) -> Delay/1(In1)
  In4/1 -> Input/4(In4)
  initial/1(Out1) -> Min_index/1(dout_sub), Out1/1
  initial/3(Out3) -> min_distance/1(In1)
  In3/1 -> Input/3(In3)
  In2/1 -> Input/2(In2)
  initial/4(Out4) -> min_distance/4(In4)
  initial/2(Out2) -> Min_index/2(doutsp_sub)
  Min_index/2(min_index_sub) -> Delay/2(In2), initial/1(In1)
  Delay/2(Out2) -> min_distance/3(In3)
  Delay/1(Out1) -> min_distance/2(In2)
  In1/1 -> Input/1(In1)
  Input/3(Out3) -> min_distance/7(In7)
  Input/4(Out4) -> min_distance/8(In8)

== system Dijkstra_Optimization_2/Dijkstra/Subsystem6 ==
  In1 : Inport
  In2 : Inport  Port=2
  Add2 : shlslibv1/Math Functions/Add  syn_add_opr=++  syn_out_f=Full Precision  syn_out_wl=16  syn_out_fl=8  syn_out_dt=signed  syn_out_sat=off  syn_out_rnd=Floor (Truncate)  synBlockType=primitive  synLatency=0  synBlockId=96  syn_sum_of_rows=off  syn_inh_port=off  syn_inh_st=on  syn_inh_stf=1  syn_en_pipe=off  syn_pipe_stg=syn_max_pipeline  syn_flow_ctrl=off
  Constant2 : shlslibv1/Sources/Constant  syn_cst_val=1  syn_cst_format=Automatic  syn_cst_wl=1  syn_cst_fl=0  syn_cst_dt=unsigned  syn_cst_rnd=on  syn_cst_st=-1  synBlockType=primitive  synLatency=0  synBlockId=15
  Switch1 : shlslibv1/Signal Operations/Switch  switchCriteria=u2 != Threshold  switchThresh=0  synBlockType=custom  synLatency=0
  min4 : shlslibv1/Memories/Delay  syn_delay_val=1  synBlockType=primitive  synLatency=1  synBlockId=104
  min5 : shlslibv1/Memories/Delay  syn_delay_val=30  synBlockType=primitive  synLatency=30  synBlockId=104
  Out1 : Outport
  wires:
  Add2/1 -> Out1/1
  In1/1 -> Add2/2
  min4/1 -> Switch1/1
  Switch1/1 -> min4/1, Add2/1
  min5/1 -> Switch1/2
  Constant2/1 -> min5/1
  In2/1 -> Switch1/3

== system Dijkstra_Optimization_2/Dijkstra/Subsystem7 ==
  In1 : Inport
  In2 : Inport  Port=2
  Add3 : shlslibv1/Math Functions/Add  syn_add_opr=++  syn_out_f=Full Precision  syn_out_wl=16  syn_out_fl=8  syn_out_dt=signed  syn_out_sat=off  syn_out_rnd=Floor (Truncate)  synBlockType=primitive  synLatency=0  synBlockId=96  syn_sum_of_rows=off  syn_inh_port=off  syn_inh_st=on  syn_inh_stf=1  syn_en_pipe=off  syn_pipe_stg=syn_max_pipeline  syn_flow_ctrl=off
  Constant4 : shlslibv1/Sources/Constant  syn_cst_val=1  syn_cst_format=Automatic  syn_cst_wl=1  syn_cst_fl=0  syn_cst_dt=unsigned  syn_cst_rnd=on  syn_cst_st=-1  synBlockType=primitive  synLatency=0  synBlockId=15
  Switch2 : shlslibv1/Signal Operations/Switch  switchCriteria=u2 != Threshold  switchThresh=0  synBlockType=custom  synLatency=0
  min6 : shlslibv1/Memories/Delay  syn_delay_val=1  synBlockType=primitive  synLatency=1  synBlockId=104
  min7 : shlslibv1/Memories/Delay  syn_delay_val=31  synBlockType=primitive  synLatency=31  synBlockId=104
  Out1 : Outport
  wires:
  Add3/1 -> Out1/1
  In2/1 -> Add3/2
  min6/1 -> Switch2/1
  Switch2/1 -> min6/1, Add3/1
  min7/1 -> Switch2/2
  Constant4/1 -> min7/1
  In1/1 -> Switch2/3

== system Dijkstra_Optimization_2/Dijkstra/Subsystem8 ==
  In1 : Inport
  Constant3 : shlslibv1/Sources/Constant  syn_cst_val=1  syn_cst_format=Automatic  syn_cst_wl=1  syn_cst_fl=0  syn_cst_dt=unsigned  syn_cst_rnd=on  syn_cst_st=-1  synBlockType=primitive  synLatency=0  synBlockId=15
  Switch6 : shlslibv1/Signal Operations/Switch  switchCriteria=u2 == Threshold  switchThresh=0  synBlockType=custom  synLatency=0
  To Workspace5 : ToWorkspace  VariableName=dist2  SaveFormat=Structure With Time  SampleTime=-1
      settings: Save2DSignal=2-D array (concatenate along first dimension)
  dist8 : shlslibv1/Sources/Sequence  syn_seq_vec=[0 1 2 3]  syn_seq_wl=4  syn_seq_fl=0  syn_seq_dt=unsigned  syn_rst_port=off  syn_en_port=off  syn_seq_st=1/(4e6)  synBlockType=custom  synLatency=1
  min1 : shlslibv1/Memories/Delay  syn_delay_val=30  synBlockType=primitive  synLatency=30  synBlockId=104
  min12 : shlslibv1/Memories/Delay  syn_delay_val=33  synBlockType=primitive  synLatency=33  synBlockId=104
  Out1 : Outport
  Out2 : Outport  Port=2
  wires:
  Constant3/1 -> min12/1
  min12/1 -> Switch6/2, Switch6/1
  Switch6/1 -> Out1/1
  min1/1 -> Out2/1, To Workspace5/1
  dist8/1 -> min1/1
  In1/1 -> Switch6/3

== system Dijkstra_Optimization_2/Dijkstra/Subsystem9 ==
  In1 : Inport
  In2 : Inport  Port=2
  In3 : Inport  Port=3
  In4 : Inport  Port=4
  In5 : Inport  Port=5
  Port In{21..24} (4 alike) : shlslibv1/Ports & Subsystems/Port In  syn_out_wl=50  syn_out_fl=0  syn_out_dt=unsigned  syn_out_st=1/(4e6)  syn_capture=on  syn_register=on  syn_out_sat=off  syn_out_rnd=on  synBlockType=port  synLatency=1  synBlockId=0
  Subsystem10 : Subsystem
  Subsystem13 : Subsystem
  Out1 : Outport
  wires:
  Port In23/1 -> Subsystem10/3(In3)
  Port In21/1 -> Subsystem10/1(In1)
  In1/1 -> Subsystem13/2(In2)
  In5/1 -> Port In24/1
  Subsystem10/1(Out1) -> Subsystem13/1(In1)
  Subsystem13/1(Out1) -> Out1/1
  Port In24/1 -> Subsystem10/4(In4)
  In2/1 -> Port In21/1
  Port In22/1 -> Subsystem10/2(In2)
  In4/1 -> Port In23/1
  In3/1 -> Port In22/1

== system Dijkstra_Optimization_2/Dijkstra/Subsystem1/Delay ==
  In1 : Inport
  In2 : Inport  Port=2
  Switch10 : shlslibv1/Signal Operations/Switch  switchCriteria=u2 != Threshold  switchThresh=0  synBlockType=custom  synLatency=0
  Switch5 : shlslibv1/Signal Operations/Switch  switchCriteria=u2 != Threshold  switchThresh=0  synBlockType=custom  synLatency=0
  dist6 : shlslibv1/Sources/Sequence  syn_seq_vec=[0 0 0 1 0 0 0 0 ]  syn_seq_wl=4  syn_seq_fl=0  syn_seq_dt=unsigned  syn_rst_port=off  syn_en_port=off  syn_seq_st=1/(4e6)  synBlockType=custom  synLatency=1
  min10 : shlslibv1/Memories/Delay  syn_delay_val=2  synBlockType=primitive  synLatency=2  synBlockId=104
  min4 : shlslibv1/Memories/Delay  syn_delay_val=1  synBlockType=primitive  synLatency=1  synBlockId=104
  min9 : shlslibv1/Memories/Delay  syn_delay_val=1  synBlockType=primitive  synLatency=1  synBlockId=104
  Out1 : Outport
  Out2 : Outport  Port=2
  wires:
  In2/1 -> Switch5/1
  dist6/1 -> min10/1
  min10/1 -> Switch5/2, Switch10/2
  In1/1 -> Switch10/1
  Switch10/1 -> Out1/1, min9/1
  Switch5/1 -> min4/1
  min9/1 -> Switch10/3
  min4/1 -> Switch5/3, Out2/1

== system Dijkstra_Optimization_2/Dijkstra/Subsystem1/Input ==
  In1 : Inport
  In2 : Inport  Port=2
  In3 : Inport  Port=3
  In4 : Inport  Port=4
  Constant5 : shlslibv1/Sources/Constant  syn_cst_val=1  syn_cst_format=Automatic  syn_cst_wl=1  syn_cst_fl=0  syn_cst_dt=unsigned  syn_cst_rnd=on  syn_cst_st=-1  synBlockType=primitive  synLatency=0  synBlockId=15
  Constant6 : shlslibv1/Sources/Constant  syn_cst_val=0  syn_cst_format=Automatic  syn_cst_wl=1  syn_cst_fl=0  syn_cst_dt=unsigned  syn_cst_rnd=on  syn_cst_st=-1  synBlockType=primitive  synLatency=0  synBlockId=15
  Graph{0..3} (4 alike) : shlslibv1/Memories/RAM  syn_ram_depth=4  syn_read_nb=1  syn_write_nb=1  syn_rw_nb=0  syn_corereset=off  syn_localreset=off  syn_initial_val=0  syn_enable_port=off  syn_rrst_port=off  syn_renable_port=off  syn_wac=Write priorization  syn_rac=Cross-port write-first  syn_init_val=0  synBlockType=primitive  synLatency=1  synBlockId=111  syn_spec_init=on
  Switch1 : shlslibv1/Signal Operations/Switch  switchCriteria=u2 != Threshold  switchThresh=0  synBlockType=custom  synLatency=0
  dist9 : shlslibv1/Sources/Sequence  syn_seq_vec=[0 1 2 3 ]  syn_seq_wl=4  syn_seq_fl=0  syn_seq_dt=unsigned  syn_rst_port=off  syn_en_port=off  syn_seq_st=1/(4e6)  synBlockType=custom  synLatency=1
  min14 : shlslibv1/Memories/Delay  syn_delay_val=5  synBlockType=primitive  synLatency=5  synBlockId=104
  min15 : shlslibv1/Memories/Delay  syn_delay_val=5  synBlockType=primitive  synLatency=5  synBlockId=104
  Out1 : Outport
  Out2 : Outport  Port=2
  Out3 : Outport  Port=3
  Out4 : Outport  Port=4
  wires:
  Constant5/1 -> min14/1, Switch1/3
  min14/1 -> Switch1/2
  Switch1/1 -> Graph3/4, Graph2/4, Graph1/4, Graph0/4
  Constant6/1 -> Switch1/1
  In1/1 -> Graph0/3
  In2/1 -> Graph1/3
  In3/1 -> Graph2/3
  In4/1 -> Graph3/3
  dist9/1 -> min15/1, Graph3/2, Graph2/2, Graph1/2, Graph0/2
  min15/1 -> Graph2/1, Graph3/1, Graph1/1, Graph0/1
  Graph0/1 -> Out1/1
  Graph3/1 -> Out4/1
  Graph2/1 -> Out3/1
  Graph1/1 -> Out2/1

== system Dijkstra_Optimization_2/Dijkstra/Subsystem1/Min_index ==
  dout_sub : Inport
  doutsp_sub : Inport  Port=2
  Comparator1 : shlslibv1/Math Functions/Comparator  syn_comp_opr=a==b  syn_comp_const=on  syn_comp_val=0  syn_en_se=off  synBlockType=primitive  synLatency=0  synBlockId=14
  Comparator2 : shlslibv1/Math Functions/Comparator  syn_comp_opr=a<=b  syn_comp_const=off  syn_comp_val=0  syn_en_se=off  synBlockType=primitive  synLatency=0  synBlockId=14
  Constant4 : shlslibv1/Sources/Constant  syn_cst_val=64  syn_cst_format=Automatic  syn_cst_wl=1  syn_cst_fl=0  syn_cst_dt=unsigned  syn_cst_rnd=on  syn_cst_st=-1  synBlockType=primitive  synLatency=0  synBlockId=15
  Convert1 : shlslibv1/Signal Operations/Convert  syn_preshift_opr=none  syn_preshift_bits=0  syn_preshift_val=0  syn_out_f=Specify  syn_out_wl=64  syn_out_fl=0  syn_out_dt_sync=unsigned  syn_out_sat=off  syn_out_rnd=Floor (Truncate)  syn_inh_port=off  syn_inh_st=off  syn_inh_stf=1  syn_en_pipe=off  syn_pipe_stg=syn_max_pipeline  syn_flow_ctrl=off  syn_sat_op=off  synBlockType=primitive  synLatency=0  synBlockId=4
  Convert2 : shlslibv1/Signal Operations/Convert  syn_preshift_opr=none  syn_preshift_bits=0  syn_preshift_val=0  syn_out_f=Specify  syn_out_wl=4  syn_out_fl=0  syn_out_dt_sync=unsigned  syn_out_sat=off  syn_out_rnd=Floor (Truncate)  syn_inh_port=off  syn_inh_st=off  syn_inh_stf=1  syn_en_pipe=off  syn_pipe_stg=syn_max_pipeline  syn_flow_ctrl=off  syn_sat_op=off  synBlockType=primitive  synLatency=0  synBlockId=4
  Mux : shlslibv1/Signal Operations/Mux  syn_in_nb=2  syn_out_f=Full Precision  syn_out_wl=11  syn_out_fl=52  syn_out_dt=unsigned  syn_en_se=off  synBlockType=primitive  synLatency=0  synBlockId=16
  Switch7 : shlslibv1/Signal Operations/Switch  switchCriteria=u2 != Threshold  switchThresh=0  synBlockType=custom  synLatency=0
  dist10 : shlslibv1/Sources/Sequence  syn_seq_vec=[1 0 0 0 ]  syn_seq_wl=4  syn_seq_fl=0  syn_seq_dt=unsigned  syn_rst_port=off  syn_en_port=off  syn_seq_st=1/(4e6)  synBlockType=custom  synLatency=1
  dist9 : shlslibv1/Sources/Sequence  syn_seq_vec=[0 1 2 3]  syn_seq_wl=4  syn_seq_fl=0  syn_seq_dt=unsigned  syn_rst_port=off  syn_en_port=off  syn_seq_st=1/(4e6)  synBlockType=custom  synLatency=1
  min : shlslibv1/Signal Operations/Mux  syn_in_nb=2  syn_out_f=Full Precision  syn_out_wl=11  syn_out_fl=52  syn_out_dt=unsigned  syn_en_se=off  synBlockType=primitive  synLatency=0  synBlockId=16
  min3 : shlslibv1/Memories/Delay  syn_delay_val=2  synBlockType=primitive  synLatency=2  synBlockId=104
  min4 : shlslibv1/Memories/Delay  syn_delay_val=1  synBlockType=primitive  synLatency=1  synBlockId=104
  min5 : shlslibv1/Memories/Delay  syn_delay_val=1  synBlockType=primitive  synLatency=1  synBlockId=104
  min6 : shlslibv1/Memories/Delay  syn_delay_val=2  synBlockType=primitive  synLatency=2  synBlockId=104
  min_index : shlslibv1/Signal Operations/Mux  syn_in_nb=2  syn_out_f=Full Precision  syn_out_wl=11  syn_out_fl=52  syn_out_dt=unsigned  syn_en_se=off  synBlockType=primitive  synLatency=0  synBlockId=16
  min_sub : Outport
  min_index_sub : Outport  Port=2
  wires:
  min3/1 -> min_index/3
  Comparator1/1 -> Mux/3
  Mux/1 -> Convert2/1
  min/1 -> Convert1/1, min_sub/1
  min_index/1 -> min_index_sub/1, min5/1
  dist9/1 -> min3/1
  dist10/1 -> min6/1
  dout_sub/1 -> Comparator2/1, min/3
  doutsp_sub/1 -> Comparator1/1
  min5/1 -> min_index/2
  Constant4/1 -> Switch7/1
  min6/1 -> Switch7/2
  Switch7/1 -> min/2, Comparator2/2
  min4/1 -> Switch7/3
  Convert2/1 -> min/1, min_index/1
  Convert1/1 -> min4/1
  Comparator2/1 -> Mux/2, Mux/1

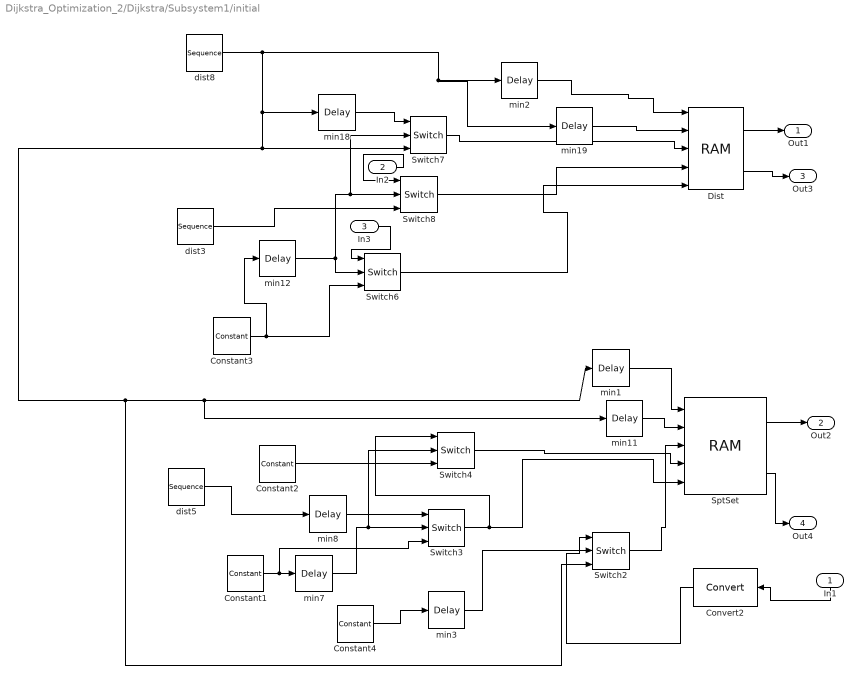
== system Dijkstra_Optimization_2/Dijkstra/Subsystem1/initial ==
  In1 : Inport
  In2 : Inport  Port=2
  In3 : Inport  Port=3
  Constant1 : shlslibv1/Sources/Constant  syn_cst_val=1  syn_cst_format=Automatic  syn_cst_wl=1  syn_cst_fl=0  syn_cst_dt=unsigned  syn_cst_rnd=on  syn_cst_st=-1  synBlockType=primitive  synLatency=0  synBlockId=15
  Constant2 : shlslibv1/Sources/Constant  syn_cst_val=0  syn_cst_format=Automatic  syn_cst_wl=1  syn_cst_fl=0  syn_cst_dt=unsigned  syn_cst_rnd=on  syn_cst_st=-1  synBlockType=primitive  synLatency=0  synBlockId=15
  Constant3 : shlslibv1/Sources/Constant  syn_cst_val=1  syn_cst_format=Automatic  syn_cst_wl=1  syn_cst_fl=0  syn_cst_dt=unsigned  syn_cst_rnd=on  syn_cst_st=-1  synBlockType=primitive  synLatency=0  synBlockId=15
  Constant4 : shlslibv1/Sources/Constant  syn_cst_val=1  syn_cst_format=Automatic  syn_cst_wl=1  syn_cst_fl=0  syn_cst_dt=unsigned  syn_cst_rnd=on  syn_cst_st=-1  synBlockType=primitive  synLatency=0  synBlockId=15
  Convert2 : shlslibv1/Signal Operations/Convert  syn_preshift_opr=none  syn_preshift_bits=0  syn_preshift_val=0  syn_out_f=Specify  syn_out_wl=4  syn_out_fl=0  syn_out_dt_sync=unsigned  syn_out_sat=off  syn_out_rnd=Floor (Truncate)  syn_inh_port=off  syn_inh_st=off  syn_inh_stf=1  syn_en_pipe=off  syn_pipe_stg=syn_max_pipeline  syn_flow_ctrl=off  syn_sat_op=off  synBlockType=primitive  synLatency=0  synBlockId=4
  "Dist " : shlslibv1/Memories/RAM  syn_ram_depth=4  syn_read_nb=2  syn_write_nb=1  syn_rw_nb=0  syn_corereset=off  syn_localreset=off  syn_initial_val=0  syn_enable_port=off  syn_rrst_port=off  syn_renable_port=off  syn_wac=Write priorization  syn_rac=Cross-port write-first  syn_init_val=0  synBlockType=primitive  synLatency=1  synBlockId=111  syn_spec_init=on
  SptSet : shlslibv1/Memories/RAM  syn_ram_depth=4  syn_read_nb=2  syn_write_nb=1  syn_rw_nb=0  syn_corereset=off  syn_localreset=off  syn_initial_val=0  syn_enable_port=off  syn_rrst_port=off  syn_renable_port=off  syn_wac=Write priorization  syn_rac=Cross-port write-first  syn_init_val=0  synBlockType=primitive  synLatency=1  synBlockId=111  syn_spec_init=on
  Switch{2..4,6..8} (6 alike) : shlslibv1/Signal Operations/Switch  switchCriteria=u2 != Threshold  switchThresh=0  synBlockType=custom  synLatency=0
  dist3 : shlslibv1/Sources/Sequence  syn_seq_vec=[0 64 64 64]  syn_seq_wl=100  syn_seq_fl=0  syn_seq_dt=unsigned  syn_rst_port=off  syn_en_port=off  syn_seq_st=1/(4e6)  synBlockType=custom  synLatency=1
  dist5 : shlslibv1/Sources/Sequence  syn_seq_vec=[0 0 0 1 0 0 0 0 ]  syn_seq_wl=4  syn_seq_fl=0  syn_seq_dt=unsigned  syn_rst_port=off  syn_en_port=off  syn_seq_st=1/(4e6)  synBlockType=custom  synLatency=1
  dist8 : shlslibv1/Sources/Sequence  syn_seq_vec=[0 1 2 3]  syn_seq_wl=4  syn_seq_fl=0  syn_seq_dt=unsigned  syn_rst_port=off  syn_en_port=off  syn_seq_st=1/(4e6)  synBlockType=custom  synLatency=1
  min1 : shlslibv1/Memories/Delay  syn_delay_val=1  synBlockType=primitive  synLatency=1  synBlockId=104
  min{3,7,11..12,19} (5 alike) : shlslibv1/Memories/Delay  syn_delay_val=5  synBlockType=primitive  synLatency=5  synBlockId=104
  min18 : shlslibv1/Memories/Delay  syn_delay_val=6  synBlockType=primitive  synLatency=6  synBlockId=104
  min2 : shlslibv1/Memories/Delay  syn_delay_val=1  synBlockType=primitive  synLatency=1  synBlockId=104
  min8 : shlslibv1/Memories/Delay  syn_delay_val=2  synBlockType=primitive  synLatency=2  synBlockId=104
  Out1 : Outport
  Out2 : Outport  Port=2
  Out3 : Outport  Port=3
  Out4 : Outport  Port=4
  wires:
  In1/1 -> Convert2/1
  In3/1 -> Switch6/1
  In2/1 -> Switch8/1
  min1/1 -> SptSet/1
  min2/1 -> "Dist "/1
  "Dist "/1 -> Out1/1
  SptSet/1 -> Out2/1
  min3/1 -> Switch2/2
  Switch4/1 -> SptSet/4
  Convert2/1 -> Switch2/1
  dist8/1 -> Switch7/3, Switch2/3, min11/1, min1/1, min18/1, min19/1, min2/1
  Constant1/1 -> Switch3/3, min7/1
  Switch3/1 -> Switch4/1, SptSet/5
  Constant2/1 -> Switch4/3
  min7/1 -> Switch4/2, Switch3/2
  dist5/1 -> min8/1
  min8/1 -> Switch3/1
  Switch2/1 -> SptSet/3
  min11/1 -> SptSet/2
  min12/1 -> Switch6/2, Switch8/2, Switch7/2
  Constant3/1 -> Switch6/3, min12/1
  Switch6/1 -> "Dist "/5
  dist3/1 -> Switch8/3
  Switch8/1 -> "Dist "/4
  min18/1 -> Switch7/1
  Switch7/1 -> "Dist "/3
  min19/1 -> "Dist "/2
  Constant4/1 -> min3/1
  SptSet/2 -> Out4/1
  "Dist "/2 -> Out3/1
